simulink model "sampleModel378"  (R2021b)
settings: Solver=VariableStepAuto  StartTime=0.0  StopTime=10.0  RelTol=1e-3
undefined symbols (not defined in the file or in its folder): Newton, Raphson
libraries: simulink x9, slpidlib x2
settings Model: Creator=user  LastModifiedBy=user

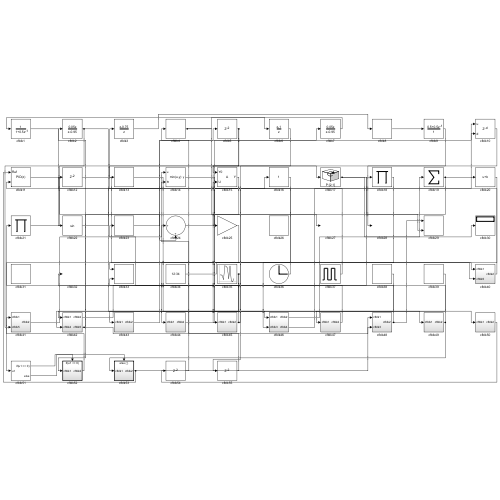
[thumbnail: Simulink's stored preview of the top-level diagram]
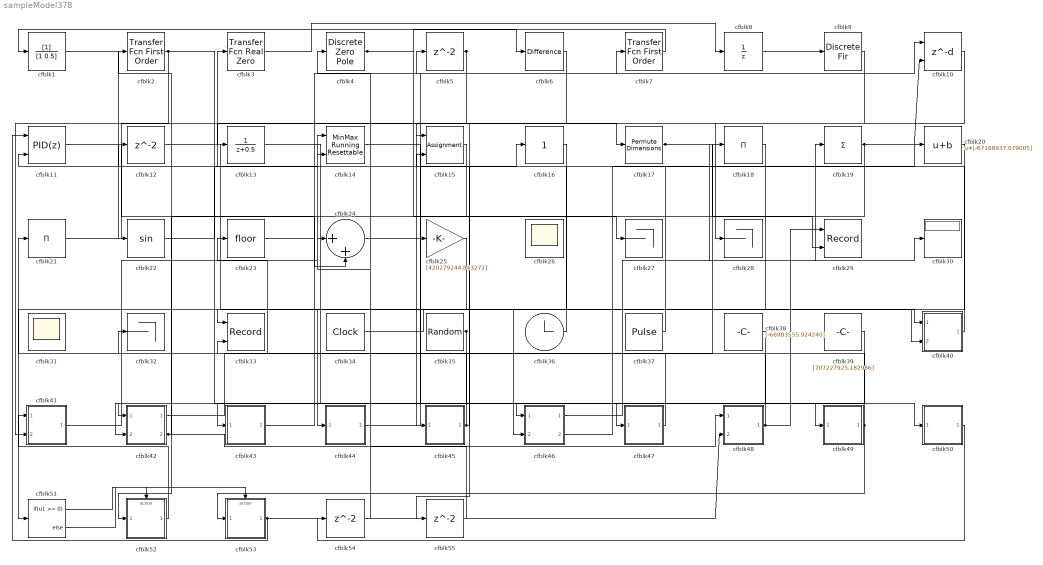
== system sampleModel378 ==
  cfblk1 : DiscreteFilter  SampleTime=1
  cfblk10 : Delay  DelayLengthSource=Input port  SampleTime=1
      settings: InputPortMap=u0,p1
  cfblk11 : slpidlib/PID Controller (2DOF)  Controller=PID  Form=Parallel  TimeDomain=Discrete-time  UseExternalTs=off  SampleTime=1  IntegratorMethod=Forward Euler  FilterMethod=Forward Euler  ControllerParametersSource=internal  P=1  I=1  D=0  UseFilter=on  N=100  b=1  c=1  TunerSelectOption=Transfer Function Based (PID Tuner App)  InitialConditionSource=internal  InitialConditionForIntegrator=0  InitialConditionForFilter=0  DifferentiatorICPrevScaledInput=0  ExternalReset=none  TrackingMode=off  Kt=1  LimitOutput=off  SatLimitsSource=internal  UpperSaturationLimit=inf  LowerSaturationLimit=-inf  LinearizeAsGain=off  AntiWindupMode=none  Kb=1  POutMin=[]  POutMax=[]  IOutMin=[]  IOutMax=[]  DOutMin=[]  DOutMax=[]  NOutMin=[]  NOutMax=[]  bOutMin=[]  bOutMax=[]  cOutMin=[]  cOutMax=[]  SumOutMin=[]  SumOutMax=[]  SaturationOutMin=[]  SaturationOutMax=[]  PParamMin=[]  PParamMax=[]  IParamMin=[]  IParamMax=[]  DParamMin=[]  DParamMax=[]  NParamMin=[]  NParamMax=[]  bParamMin=[]  bParamMax=[]  cParamMin=[]  cParamMax=[]  KbParamMin=[]  KbParamMax=[]  KtParamMin=[]  KtParamMax=[]  KbOutMin=[]  KbOutMax=[]  KtOutMin=[]  KtOutMax=[]  IntegratorOutMin=[]  IntegratorOutMax=[]  FilterOutMin=[]  FilterOutMax=[]  SumI1OutMin=[]  SumI1OutMax=[]  SumI2OutMin=[]  SumI2OutMax=[]  SumI3OutMin=[]  SumI3OutMax=[]  SumI4OutMin=[]  SumI4OutMax=[]  SumDOutMin=[]  SumDOutMax=[]  Sum1OutMin=[]  Sum1OutMax=[]  Sum2OutMin=[]  Sum2OutMax=[]  Sum3OutMin=[]  Sum3OutMax=[]  DifferentiatorOutMin=[]  DifferentiatorOutMax=[]  FilterDiffOutCoefMin=[]  FilterDiffOutCoefMax=[]  ReciprocalOutMin=[]  ReciprocalOutMax=[]  SumDenOutMin=[]  SumDenOutMax=[]  SumNumOutMin=[]  SumNumOutMax=[]  DivideOutMin=[]  DivideOutMax=[]  UdiffTsProdOutMin=[]  UdiffTsProdOutMax=[]  NTsProdOutMin=[]  NTsProdOutMax=[]  UintegralTsProdOutMin=[]  UintegralTsProdOutMax=[]  UngainTsProdOutMin=[]  UngainTsProdOutMax=[]  IntegratorContinuousStateAttributes=''  IntegratorStateMustResolveToSignalObject=off  IntegratorRTWStateStorageClass=Auto  FilterContinuousStateAttributes=''  FilterStateMustResolveToSignalObject=off  FilterRTWStateStorageClass=Auto  ParallelPVariant=InternalParameters  IdealPVariant=Disabled  IVariant=InternalParameters  DVariant=InternalParameters  bVariant=InternalParameters  cVariant=InternalParameters  IntegratorVariant=Discrete  SatVariant=Disabled  AWVariant=Passthrough  PCopyVariant=Disabled  TRVariant=Disabled  FdbkBlocksVariant=Forward  IdealPFdbkVariant=Disabled  SatFdbkVariant=Disabled  DerivativeFilterVariant=ForwardEulerFilter  NVariant=InternalParameters  NCopyVariant=Disabled  FilterICVariant=InternalICsFilter  IntegratorICVariant=InternalICs  ExternalResetVariant=Disabled  TRSumVariant=Passthrough  SumFdbkVariant=Disabled  SumVariant=Sum_PID  TsampFilterVariant=InternalTs  TsampNgainVariant=Passthrough  TsampIntegralVariant=Passthrough  ExternalSaturationOutDataTypeStr=Inherit: Same as second input
      settings: SourceProductBaseCode=SL
  cfblk{5,12,54..55} (4 alike) : Delay  SampleTime=1
  cfblk13 : DiscreteTransferFcn  SampleTime=1
  cfblk14 : simulink/Math Operations/MinMax Running Resettable  Function=min  vinit=0.0
  cfblk15 : Assignment  DiagnosticForDimensions=Warning  IndexOptions=Index vector (dialog)  Indices=1  OutputSizes=1
  cfblk16 : simulink/Math Operations/Slider Gain  gain=1  low=0  high=2
  cfblk17 : PermuteDimensions
  cfblk18 : Product  Inputs=*
  cfblk19 : Sum  Inputs=+
  cfblk2 : simulink/Discrete/Transfer Fcn First Order  PoleZ=0.95  ICPrevOutput=0.0  DoSatur=off
  cfblk20 : Bias  Bias=[-67168937.079005]
  cfblk21 : Product  Inputs=*
  cfblk22 : Trigonometry
  cfblk23 : Rounding
  cfblk24 : Sum  Inputs=|++
  cfblk25 : Gain  Gain=[420279244.843272]
  cfblk26 : Scope
      settings: Floating=on
  cfblk27 : Terminator
  cfblk28 : Terminator
  cfblk29 : Record  FileSettingsInternal="{\"entries\":[{\"content\":{\"excelSettings\":{\"content\":{},\"type\":\"Streamout.ExcelSettings\"}},\"type\":\"Streamout.FileSettingStorage\",\"uuid\":\"6df36993-1ca7-4f53-a27a-4bab49cf4c4d\"}],\"packageUris\":[\"http://schema.mathworks.com/mf0/streamout_blocks/R2020a\"],\"version\":\"1.0\"}"  Layout=[1 1]  SignalsInternal="{\"entries\":[{\"content\":{\"signals\":[{\"content\":{\"blockPath\":[\"sampleModel378/cfblk29\"],\"channel\":[],\"dimensions\":[1],\"domain\":\"sampleModel378/cfblk29\",\"lineColor\":\"#a2142f\",\"plots\":[1],\"port\":1,\"sid\":[\"\"],\"signalID\":15645,\"signalName\":\"cfblk48\"},\"type\":\"RecordBlkView.Signal\",\"uuid\":\"b7a92434-58dd-484f-9ae9-0947a41cb0fb\"},{\"content\":{\"blockPath\":[\"sampleModel378/cfblk29\"],\"channel\":[],\"dimensions\":[1,1],\"domain\":\"sampleModel378/cfblk29\",\"lineColor\":\"#139fff\",\"plots\":[1],\"port\":2,\"sid\":[\"\"],\"signalID\":15649,\"signalName\":\"cfblk17\"},\"type\":\"RecordBlkView.Signal\",\"uuid\":\"686b212e-d350-46b9-a4ee-f4e566e25235\"}]},\"type\":\"RecordBlkView.InputSignals\",\"uuid\":\"cb0ce280-3bd0-4488-938b-a44a3a88da29\"}],\"packageUris\":[\"http://schema.mathworks.com/mf0/streamout_blocks/R2020a\"],\"version\":\"1.0\"}"  VisualizationBindings="{\"xyplotplugin\":{\"info\":[{\"series\":[{\"bindingParametersList\":[{\"parameter\":\"X-Axis\",\"signalID\":15645,\"signalName\":\"cfblk48\"},{\"parameter\":\"Y-Axis\",\"signalID\":15649,\"signalName\":\"cfblk17\"}],\"seriesID\":14617}],\"subplotID\":1}]}}"  CompatibilityTag=XY
  cfblk3 : simulink/Discrete/Transfer Fcn Real Zero  ZeroZ=0.75  ICPrevInput=0.0  DoSatur=off
      settings: SourceProductBaseCode=SL
  cfblk30 : Display
  cfblk31 : Scope
      settings: Floating=on
  cfblk32 : Terminator
  cfblk33 : Record  FileSettingsInternal="{\"entries\":[{\"content\":{\"excelSettings\":{\"content\":{},\"type\":\"Streamout.ExcelSettings\"}},\"type\":\"Streamout.FileSettingStorage\",\"uuid\":\"73c6cb0a-a20f-415f-bd31-4637980e3ec7\"}],\"packageUris\":[\"http://schema.mathworks.com/mf0/streamout_blocks/R2020a\"],\"version\":\"1.0\"}"  Layout=[1 1]  SignalsInternal="{\"entries\":[{\"content\":{\"signals\":[{\"content\":{\"blockPath\":[\"sampleModel378/cfblk33\"],\"channel\":[],\"dimensions\":[1],\"domain\":\"sampleModel378/cfblk33\",\"lineColor\":\"#a2142f\",\"plots\":[1],\"port\":1,\"sid\":[\"\"],\"signalID\":15653,\"signalName\":\"cfblk20\"},\"type\":\"RecordBlkView.Signal\",\"uuid\":\"f24bfdf5-7cfe-4500-ad8e-d3e3a512e165\"},{\"content\":{\"blockPath\":[\"sampleModel378/cfblk33\"],\"channel\":[],\"dimensions\":[1],\"domain\":\"sampleModel378/cfblk33\",\"lineColor\":\"#139fff\",\"plots\":[1],\"port\":2,\"sid\":[\"\"],\"signalID\":15657,\"signalName\":\"cfblk49\"},\"type\":\"RecordBlkView.Signal\",\"uuid\":\"106fbb2d-dc0e-417f-9497-bac0c250f028\"}]},\"type\":\"RecordBlkView.InputSignals\",\"uuid\":\"a0857859-61ff-4942-8b4c-76f88fc253a8\"}],\"packageUris\":[\"http://schema.mathworks.com/mf0/streamout_blocks/R2020a\"],\"version\":\"1.0\"}"  VisualizationBindings="{\"xyplotplugin\":{\"info\":[{\"series\":[{\"bindingParametersList\":[{\"parameter\":\"X-Axis\",\"signalID\":15653,\"signalName\":\"cfblk20\"},{\"parameter\":\"Y-Axis\",\"signalID\":15657,\"signalName\":\"cfblk49\"}],\"seriesID\":9810}],\"subplotID\":1}]}}"  CompatibilityTag=XY
  cfblk34 : DigitalClock
  cfblk35 : RandomNumber  Mean=[27584.503677]  Variance=[23287.173780]  Seed=[558490118.000000]  SampleTime=0.1
  cfblk36 : Clock
  cfblk37 : DiscretePulseGenerator  PulseType=Time based  Amplitude=[110338320.501734]  Period=[47659545.084491]  PulseWidth=5  PhaseDelay=[8.000000]
  cfblk38 : Constant  Value=[-66983555.924240]  SampleTime=1
  cfblk39 : Constant  Value=[707227925.182986]  SampleTime=1
  cfblk4 : DiscreteZeroPole  Poles=[0 0.5]  Gain=1
  cfblk40 : Subsystem
  cfblk41 : Subsystem
  cfblk42 : Subsystem
  cfblk43 : Subsystem
  cfblk44 : Subsystem
  cfblk45 : Subsystem
  cfblk46 : Subsystem
  cfblk47 : Subsystem
  cfblk48 : Subsystem
  cfblk49 : Subsystem
  cfblk50 : Subsystem
  cfblk51 : If  IfExpression=u1 >= 0  SampleTime=1
  cfblk52 : Subsystem  TreatAsAtomicUnit=on
  cfblk53 : Subsystem  TreatAsAtomicUnit=on
  cfblk6 : simulink/Discrete/Difference  ICPrevInput=0.0  OutMin=[]  OutMax=[]  OutDataTypeStr=Inherit: Inherit via back propagation  OutDataType=fixdt(1, 16)  OutScaling=2^-10  DoSatur=off
  cfblk7 : simulink/Discrete/Transfer Fcn First Order  PoleZ=0.95  ICPrevOutput=0.0  DoSatur=off
  cfblk8 : UnitDelay  HasFrameUpgradeWarning=on
  cfblk9 : DiscreteFir  SampleTime=1
  wires:
  cfblk20/1 -> cfblk33/1
  cfblk44/1(cfblk2) -> cfblk16/1
  cfblk34/1 -> cfblk40/1(cfblk1)
  cfblk21/1 -> cfblk17/1
  cfblk5/1 -> cfblk45/1(cfblk1), cfblk15/1
  cfblk1/1 -> cfblk22/1
  cfblk41/1(cfblk2) -> cfblk14/1
  cfblk37/1 -> cfblk3/1
  cfblk13/1 -> cfblk50/1(cfblk1)
  cfblk16/1 -> cfblk51/1
  cfblk25/1 -> cfblk44/1(cfblk1)
  cfblk12/1 -> cfblk40/2(cfblk5)
  cfblk9/1 -> cfblk28/1
  cfblk53/1(cfblk2) -> cfblk11/1, cfblk48/2(cfblk3)
  cfblk17/1 -> cfblk30/1, cfblk29/2
  cfblk8/1 -> cfblk9/1
  cfblk35/1 -> cfblk42/1(cfblk1), cfblk43/1(cfblk1)
  cfblk23/1 -> cfblk5/1
  cfblk47/1(cfblk2) -> cfblk23/1
  cfblk24/1 -> cfblk10/1
  cfblk2/1 -> cfblk46/1(cfblk1), cfblk41/2(cfblk5)
  cfblk42/1(cfblk2) -> cfblk18/1
  cfblk38/1 -> cfblk42/2(cfblk4)
  cfblk52/1(cfblk2) -> cfblk41/1(cfblk1)
  cfblk11/1 -> cfblk24/2
  cfblk10/1 -> cfblk13/1
  cfblk49/1(cfblk2) -> cfblk53/1(cfblk1), cfblk33/2
  cfblk3/1 -> cfblk8/1
  cfblk46/1(cfblk2) -> cfblk19/1
  cfblk43/1(cfblk2) -> cfblk7/1
  cfblk40/1(cfblk2) -> cfblk11/2
  cfblk39/1 -> cfblk47/1(cfblk1)
  cfblk19/1 -> cfblk10/2, cfblk25/1
  cfblk45/1(cfblk2) -> cfblk12/1, cfblk15/2
  cfblk22/1 -> cfblk14/2
  cfblk46/2(cfblk4) -> cfblk20/1
  cfblk36/1 -> cfblk2/1
  cfblk42/2(cfblk5) -> cfblk32/1, cfblk48/1(cfblk1)
  cfblk48/1(cfblk2) -> cfblk21/1, cfblk29/1
  cfblk15/1 -> cfblk52/1(cfblk1)
  cfblk18/1 -> cfblk46/2(cfblk3)
  cfblk14/1 -> cfblk49/1(cfblk1)
  cfblk7/1 -> cfblk1/1
  cfblk4/1 -> cfblk27/1, cfblk6/1
  cfblk51/1 -> cfblk52/Action
  cfblk51/2 -> cfblk53/Action
  cfblk50/1(cfblk2) -> cfblk54/1
  cfblk54/1 -> cfblk24/1
  cfblk6/1 -> cfblk55/1
  cfblk55/1 -> cfblk4/1

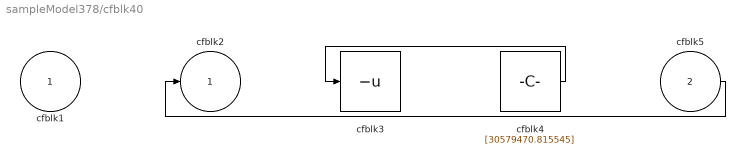
== system sampleModel378/cfblk40 ==
  cfblk1 : Inport
  cfblk5 : Inport  Port=2
  cfblk3 : UnaryMinus
  cfblk4 : Constant  Value=[30579470.815545]  SampleTime=1
  cfblk2 : Outport
  wires:
  cfblk4/1 -> cfblk3/1
  cfblk5/1 -> cfblk2/1

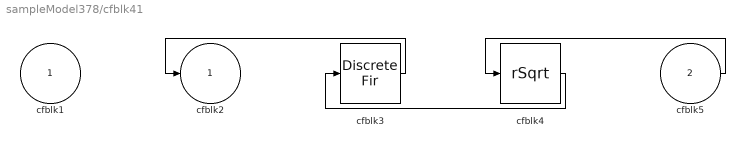
== system sampleModel378/cfblk41 ==
  cfblk1 : Inport
  cfblk5 : Inport  Port=2
  cfblk3 : DiscreteFir  SampleTime=1
  cfblk4 : Sqrt  Operator=rSqrt  AlgorithmType=Newton-Raphson  SaturateOnIntegerOverflow=on
  cfblk2 : Outport
  wires:
  cfblk3/1 -> cfblk2/1
  cfblk4/1 -> cfblk3/1
  cfblk5/1 -> cfblk4/1

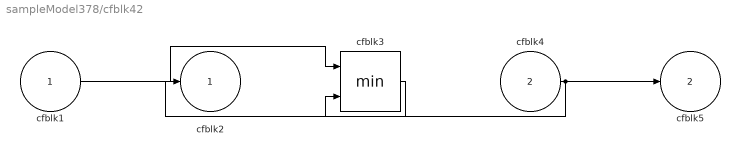
== system sampleModel378/cfblk42 ==
  cfblk1 : Inport
  cfblk4 : Inport  Port=2
  cfblk3 : MinMax  Inputs=2
  cfblk2 : Outport
  cfblk5 : Outport  Port=2
  wires:
  cfblk4/1 -> cfblk5/1, cfblk3/2
  cfblk1/1 -> cfblk3/1
  cfblk3/1 -> cfblk2/1

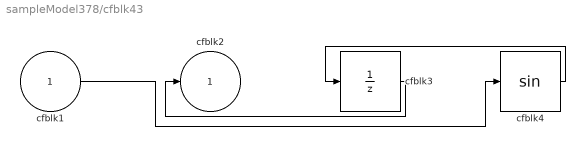
== system sampleModel378/cfblk43 ==
  cfblk1 : Inport
  cfblk3 : UnitDelay  HasFrameUpgradeWarning=on
  cfblk4 : Trigonometry
  cfblk2 : Outport
  wires:
  cfblk4/1 -> cfblk3/1
  cfblk3/1 -> cfblk2/1
  cfblk1/1 -> cfblk4/1

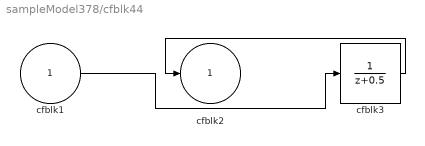
== system sampleModel378/cfblk44 ==
  cfblk1 : Inport
  cfblk3 : DiscreteTransferFcn  SampleTime=1
  cfblk2 : Outport
  wires:
  cfblk3/1 -> cfblk2/1
  cfblk1/1 -> cfblk3/1

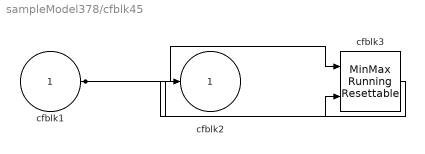
== system sampleModel378/cfblk45 ==
  cfblk1 : Inport
  cfblk3 : simulink/Math Operations/MinMax Running Resettable  Function=min  vinit=0.0
  cfblk2 : Outport
  wires:
  cfblk1/1 -> cfblk3/1, cfblk3/2
  cfblk3/1 -> cfblk2/1

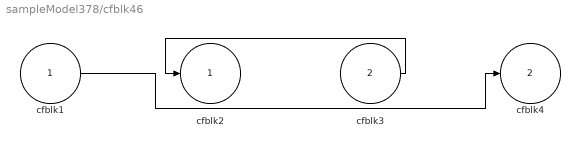
== system sampleModel378/cfblk46 ==
  cfblk1 : Inport
  cfblk3 : Inport  Port=2
  cfblk2 : Outport
  cfblk4 : Outport  Port=2
  wires:
  cfblk3/1 -> cfblk2/1
  cfblk1/1 -> cfblk4/1

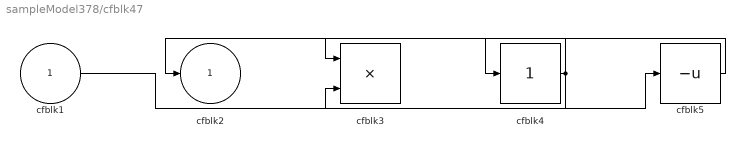
== system sampleModel378/cfblk47 ==
  cfblk1 : Inport
  cfblk3 : Product
  cfblk4 : simulink/Math Operations/Slider Gain  gain=1  low=0  high=2
  cfblk5 : UnaryMinus
  cfblk2 : Outport
  wires:
  cfblk4/1 -> cfblk2/1, cfblk3/1, cfblk3/2
  cfblk1/1 -> cfblk5/1
  cfblk5/1 -> cfblk4/1

== system sampleModel378/cfblk48 ==
  cfblk1 : Inport
  cfblk3 : Inport  Port=2
  cfblk2 : Outport
  wires:
  cfblk1/1 -> cfblk2/1

== system sampleModel378/cfblk49 ==
  cfblk1 : Inport
  cfblk3 : Gain  Gain=[-630913622.633347]
  cfblk2 : Outport
  wires:
  cfblk1/1 -> cfblk3/1
  cfblk3/1 -> cfblk2/1

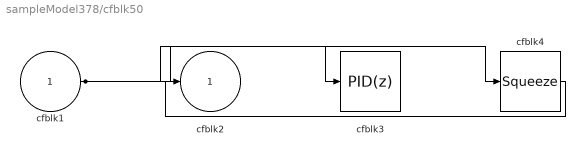
== system sampleModel378/cfblk50 ==
  cfblk1 : Inport
  cfblk3 : slpidlib/PID Controller  Controller=PID  Form=Parallel  TimeDomain=Discrete-time  UseExternalTs=off  SampleTime=1  IntegratorMethod=Forward Euler  FilterMethod=Forward Euler  ControllerParametersSource=internal  P=1  I=1  D=0  UseFilter=on  N=100  TunerSelectOption=Transfer Function Based (PID Tuner App)  InitialConditionSource=internal  InitialConditionForIntegrator=0  InitialConditionForFilter=0  DifferentiatorICPrevScaledInput=0  ExternalReset=none  TrackingMode=off  Kt=1  LimitOutput=off  SatLimitsSource=internal  UpperSaturationLimit=inf  LowerSaturationLimit=-inf  LinearizeAsGain=off  AntiWindupMode=none  Kb=1  POutMin=[]  POutMax=[]  IOutMin=[]  IOutMax=[]  DOutMin=[]  DOutMax=[]  NOutMin=[]  NOutMax=[]  SumOutMin=[]  SumOutMax=[]  SaturationOutMin=[]  SaturationOutMax=[]  PParamMin=[]  PParamMax=[]  IParamMin=[]  IParamMax=[]  DParamMin=[]  DParamMax=[]  NParamMin=[]  NParamMax=[]  KbParamMin=[]  KbParamMax=[]  KtParamMin=[]  KtParamMax=[]  KbOutMin=[]  KbOutMax=[]  KtOutMin=[]  KtOutMax=[]  IntegratorOutMin=[]  IntegratorOutMax=[]  FilterOutMin=[]  FilterOutMax=[]  SumI1OutMin=[]  SumI1OutMax=[]  SumI2OutMin=[]  SumI2OutMax=[]  SumI3OutMin=[]  SumI3OutMax=[]  SumI4OutMin=[]  SumI4OutMax=[]  SumDOutMin=[]  SumDOutMax=[]  DifferentiatorOutMin=[]  DifferentiatorOutMax=[]  FilterDiffOutCoefMin=[]  FilterDiffOutCoefMax=[]  ReciprocalOutMin=[]  ReciprocalOutMax=[]  SumDenOutMin=[]  SumDenOutMax=[]  SumNumOutMin=[]  SumNumOutMax=[]  DivideOutMin=[]  DivideOutMax=[]  UdiffTsProdOutMin=[]  UdiffTsProdOutMax=[]  NTsProdOutMin=[]  NTsProdOutMax=[]  UintegralTsProdOutMin=[]  UintegralTsProdOutMax=[]  UngainTsProdOutMin=[]  UngainTsProdOutMax=[]  IntegratorContinuousStateAttributes=''  IntegratorStateMustResolveToSignalObject=off  IntegratorRTWStateStorageClass=Auto  FilterContinuousStateAttributes=''  FilterStateMustResolveToSignalObject=off  FilterRTWStateStorageClass=Auto  ParallelPVariant=InternalParameters  IdealPVariant=Disabled  IVariant=InternalParameters  DVariant=InternalParameters  IntegratorVariant=Discrete  SatVariant=Disabled  AWVariant=Passthrough  PCopyVariant=Disabled  TRVariant=Disabled  FdbkBlocksVariant=Forward  IdealPFdbkVariant=Disabled  SatFdbkVariant=Disabled  DerivativeFilterVariant=ForwardEulerFilter  NVariant=InternalParameters  NCopyVariant=Disabled  FilterICVariant=InternalICsFilter  IntegratorICVariant=InternalICs  ExternalResetVariant=Disabled  TRSumVariant=Passthrough  SumFdbkVariant=Disabled  SumVariant=Sum_PID  TsampFilterVariant=InternalTs  TsampNgainVariant=Passthrough  TsampIntegralVariant=Passthrough  ExternalSaturationOutDataTypeStr=Inherit: Same as second input
  cfblk4 : Squeeze
  cfblk2 : Outport
  wires:
  cfblk1/1 -> cfblk4/1, cfblk3/1
  cfblk4/1 -> cfblk2/1

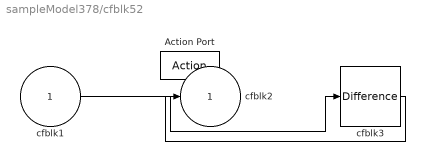
== system sampleModel378/cfblk52 ==
  cfblk1 : Inport
  Action Port : ActionPort  ActionPortLabel=if(u1 >= 0)
  cfblk3 : simulink/Discrete/Difference  ICPrevInput=0.0  OutMin=[]  OutMax=[]  OutDataTypeStr=Inherit: Inherit via back propagation  OutDataType=fixdt(1, 16)  OutScaling=2^-10  DoSatur=off
  cfblk2 : Outport
  wires:
  cfblk1/1 -> cfblk3/1
  cfblk3/1 -> cfblk2/1

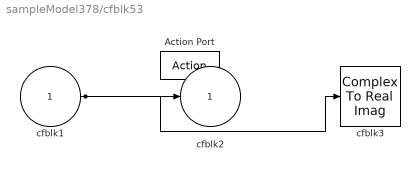
== system sampleModel378/cfblk53 ==
  cfblk1 : Inport
  Action Port : ActionPort  ActionPortLabel=else
  cfblk3 : ComplexToRealImag
  cfblk2 : Outport
  wires:
  cfblk1/1 -> cfblk2/1, cfblk3/1
